simulink model "vehicleModel"  (R2023b)
settings: Solver=VariableStepAuto  StartTime=0.0  StopTime=10.0  RelTol=1e-3
values from neighbouring files (symbols this model uses):
  b1 = b(1,:)    [bicyclekinematicmodel.m]
  b2 = b(2,:)    [bicyclekinematicmodel.m]
undefined symbols (not defined in the file or in its folder): a, linear, position
libraries: ros2lib x8, fuzblock x1
settings Model: Creator=samee  LastModifiedBy=AUVSL

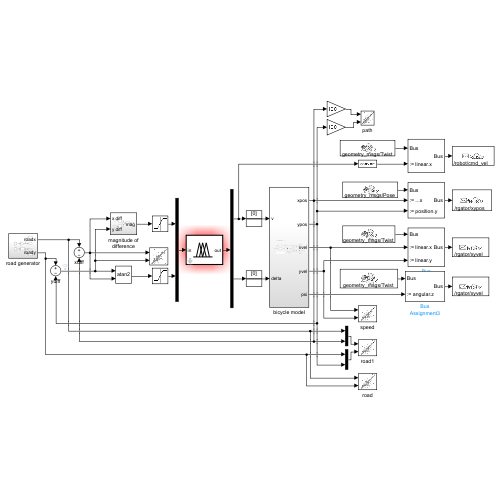
[thumbnail: Simulink's stored preview of the top-level diagram]
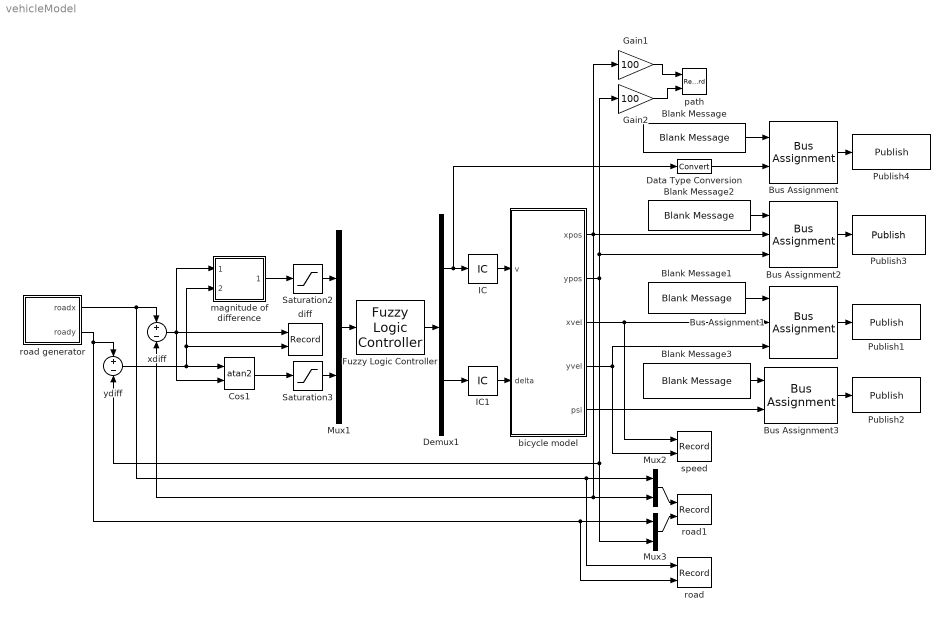
== system vehicleModel ==
  Blank Message : ros2lib/Blank Message  messageClass=Message  entityType=geometry_msgs/Twist  messageType=geometry_msgs/Twist  SampleTime=inf
  Blank Message1 : ros2lib/Blank Message  messageClass=Message  entityType=geometry_msgs/Twist  messageType=geometry_msgs/Twist  SampleTime=inf
  Blank Message2 : ros2lib/Blank Message  messageClass=Message  entityType=geometry_msgs/Pose  messageType=geometry_msgs/Pose  SampleTime=inf
  Blank Message3 : ros2lib/Blank Message  messageClass=Message  entityType=geometry_msgs/Twist  messageType=geometry_msgs/Twist  SampleTime=inf
  Bus Assignment : BusAssignment  AssignedSignals=linear.x
  Bus Assignment1 : BusAssignment  AssignedSignals=linear.x,linear.y
  Bus Assignment2 : BusAssignment  AssignedSignals=position.x,position.y
  Bus Assignment3 : BusAssignment  AssignedSignals=angular.z
  Cos1 : Trigonometry  Operator=atan2
  Data Type Conversion : DataTypeConversion  SaturateOnIntegerOverflow=off  RndMeth=Floor
  Demux1 : Demux  Outputs=2
  Fuzzy Logic Controller : fuzblock/Fuzzy Logic  Controller  FIS=fismatrix  OutputSampleNumber=101  DataType=double  FuzzifiedInputs=off  RuleFiringStrengths=off  RuleOutputs=off  AggregatedOutputs=off  SimulateUsing=Interpreted execution  OutOfRangeInputValueMessage=warning  NoRuleFiredMessage=warning  EmptyOutputFuzzySetMessage=warning
  Gain1 : Gain  Gain=100
  Gain2 : Gain  Gain=100
  IC : InitialCondition  Value=0
  IC1 : InitialCondition  Value=0
  Mux1 : Mux  Inputs=2
  Mux2 : Mux  Inputs=2
  Mux3 : Mux  Inputs=2
  Publish1 : ros2lib/Publish  topicSource=Specify your own  topic=/rgator/xyvel  messageType=geometry_msgs/Twist  QOSHistory=Keep last  QOSDepth=1  QOSReliability=Reliable  QOSDurability=Volatile
  Publish2 : ros2lib/Publish  topicSource=Specify your own  topic=/rgator/xyvel  messageType=geometry_msgs/Twist  QOSHistory=Keep last  QOSDepth=1  QOSReliability=Reliable  QOSDurability=Volatile
  Publish3 : ros2lib/Publish  topicSource=Specify your own  topic=/rgator/xypos  messageType=geometry_msgs/Pose  QOSHistory=Keep last  QOSDepth=1  QOSReliability=Reliable  QOSDurability=Volatile
  Publish4 : ros2lib/Publish  topicSource=Specify your own  topic=/robot/cmd_vel  messageType=geometry_msgs/Twist  QOSHistory=Keep last  QOSDepth=1  QOSReliability=Reliable  QOSDurability=Volatile
  Saturation2 : Saturate  UpperLimit=100  LowerLimit=0  LinearizeAsGain=off
  Saturation3 : Saturate  UpperLimit=1  LowerLimit=-1
  bicycle model : Subsystem
  diff : Record  FileSettingsInternal="{\"entries\":[{\"content\":{\"excelSettings\":{\"content\":{},\"type\":\"Streamout.ExcelSettings\"}},\"type\":\"Streamout.FileSettingStorage\",\"uuid\":\"\"}],\"packageUris\":[\"http:\\/\\/schema.mathworks.com\\/mf0\\/streamout_blocks\\/R2020a\"],\"version\":\"1.0\"}"  Layout=[1 1]  SignalsInternal="{\"entries\":[{\"content\":{\"signals\":[{\"content\":{\"blockPath\":[],\"dimensions\":[1],\"domain\":\"\",\"lineColor\":\"#edb120\",\"plots\":[ 1 ],\"port\":1,\"signalID\":1,\"signalName\":\"xdiff\"},\"type\":\"RecordBlkView.Signal\",\"uuid\":\"\"},{\"content\":{\"blockPath\":[],\"dimensions\":[1],\"domain\":\"\",\"lineColor\":\"#7e2f8e\",\"plots\":[ 1 ],\"port\":2,\"signalID\":2,\"signalName\":\"ydiff\"},\"type\":\"RecordBlkView.Signal\",\"uuid\":\"\"}]},\"type\":\"RecordBlkView.InputSignals\",\"uuid\":\"\"}],\"packageUris\":[\"http:\\/\\/schema.mathworks.com\\/mf0\\/streamout_blocks\\/R2020a\"],\"version\":\"1.0\"}"  VisualizationBindings="{\"xyplotplugin\":{\"info\":[{\"series\":[{\"bindingParametersList\":[{\"parameter\":\"X-Axis\",\"signalID\":1,\"signalName\":\"xdiff\"},{\"parameter\":\"Y-Axis\",\"signalID\":2,\"signalName\":\"ydiff\"}],\"seriesID\":0}],\"subplotID\":1}]}}"  CompatibilityTag=XY
  magnitude of difference : Subsystem
  path : Record  FileSettingsInternal="{\"entries\":[{\"content\":{\"excelSettings\":{\"content\":{},\"type\":\"Streamout.ExcelSettings\"}},\"type\":\"Streamout.FileSettingStorage\",\"uuid\":\"\"}],\"packageUris\":[\"http:\\/\\/schema.mathworks.com\\/mf0\\/streamout_blocks\\/R2020a\"],\"version\":\"1.0\"}"  Layout=[1 1]  SignalsInternal="{\"entries\":[{\"content\":{\"signals\":[{\"content\":{\"blockPath\":[],\"dimensions\":[1],\"domain\":\"\",\"lineColor\":\"#77ac30\",\"plots\":[ 1 ],\"port\":1,\"signalID\":1,\"signalName\":\"Gain\"},\"type\":\"RecordBlkView.Signal\",\"uuid\":\"\"},{\"content\":{\"blockPath\":[],\"dimensions\":[1],\"domain\":\"\",\"lineColor\":\"#4dbeee\",\"plots\":[ 1 ],\"port\":2,\"signalID\":2,\"signalName\":\"Gain1\"},\"type\":\"RecordBlkView.Signal\",\"uuid\":\"\"}]},\"type\":\"RecordBlkView.InputSignals\",\"uuid\":\"\"}],\"packageUris\":[\"http:\\/\\/schema.mathworks.com\\/mf0\\/streamout_blocks\\/R2020a\"],\"version\":\"1.0\"}"  VisualizationBindings="{\"xyplotplugin\":{\"info\":[{\"series\":[{\"bindingParametersList\":[{\"parameter\":\"X-Axis\",\"signalID\":1,\"signalName\":\"Gain\"},{\"parameter\":\"Y-Axis\",\"signalID\":2,\"signalName\":\"Gain1\"}],\"seriesID\":0}],\"subplotID\":1}]}}"  CompatibilityTag=XY
  road : Record  FileSettingsInternal="{\"entries\":[{\"content\":{\"excelSettings\":{\"content\":{},\"type\":\"Streamout.ExcelSettings\"}},\"type\":\"Streamout.FileSettingStorage\",\"uuid\":\"\"}],\"packageUris\":[\"http:\\/\\/schema.mathworks.com\\/mf0\\/streamout_blocks\\/R2020a\"],\"version\":\"1.0\"}"  Layout=[1 1]  SignalsInternal="{\"entries\":[{\"content\":{\"signals\":[{\"content\":{\"blockPath\":[],\"dimensions\":[1],\"domain\":\"\",\"lineColor\":\"#a2142f\",\"plots\":[ 1 ],\"port\":1,\"signalID\":1,\"signalName\":\"road generator:1\"},\"type\":\"RecordBlkView.Signal\",\"uuid\":\"\"},{\"content\":{\"blockPath\":[],\"dimensions\":[1],\"domain\":\"\",\"lineColor\":\"#139fff\",\"plots\":[ 1 ],\"port\":2,\"signalID\":2,\"signalName\":\"road generator:2\"},\"type\":\"RecordBlkView.Signal\",\"uuid\":\"\"}]},\"type\":\"RecordBlkView.InputSignals\",\"uuid\":\"\"}],\"packageUris\":[\"http:\\/\\/schema.mathworks.com\\/mf0\\/streamout_blocks\\/R2020a\"],\"version\":\"1.0\"}"  VisualizationBindings="{\"xyplotplugin\":{\"info\":[{\"series\":[{\"bindingParametersList\":[{\"parameter\":\"X-Axis\",\"signalID\":1,\"signalName\":\"road generator:1\"},{\"parameter\":\"Y-Axis\",\"signalID\":2,\"signalName\":\"road generator:2\"}],\"seriesID\":0}],\"subplotID\":1}]}}"  CompatibilityTag=XY
  road generator : Subsystem
  road1 : Record  FileSettingsInternal="{\"entries\":[{\"content\":{\"excelSettings\":{\"content\":{},\"type\":\"Streamout.ExcelSettings\"}},\"type\":\"Streamout.FileSettingStorage\",\"uuid\":\"\"}],\"packageUris\":[\"http:\\/\\/schema.mathworks.com\\/mf0\\/streamout_blocks\\/R2020a\"],\"version\":\"1.0\"}"  Layout=[1 1]  SignalsInternal="{\"entries\":[{\"content\":{\"signals\":[{\"content\":{\"blockPath\":[],\"dimensions\":[2],\"domain\":\"\",\"hasChildren\":true,\"lineColor\":\"#a2142f\",\"port\":1,\"signalID\":1,\"signalName\":\"Mux1\"},\"type\":\"RecordBlkView.Signal\",\"uuid\":\"\"},{\"content\":{\"blockPath\":[],\"channel\":[1],\"dimensions\":[2],\"domain\":\"\",\"lineColor\":\"#139fff\",\"parentID\":1,\"plots\":[ 1 ],\"port\":1,\"signalID\":2,\"signalName\":\"Mux1\"},\"type\":\"RecordBlkView.Signal\",\"uuid\":\"\"},{\"content\":{\"blockPath\":[],\"channel\":[2],\"dimensions\":[2],\"domain\":\"\",\"lineColor\":\"#fe330a\",\"parentID\":1,\"plots\":[ 1 ],\"port\":1,\"signalID\":3,\"signalName\":\"Mux1\"},\"type\":\"RecordBlkView.Signal\",\"uuid\":\"\"},{\"content\":{\"blockPath\":[],\"dimensions\":[2],\"domain\":\"\",\"hasChildren\":true,\"lineColor\":\"#ff6929\",\"port\":2,\"signalID\":4,\"signalName\":\"Mux2\"},\"type\":\"RecordBlkView.Signal\",\"uuid\":\"\"},{\"content\":{\"blockPath\":[],\"channel\":[1],\"dimensions\":[2],\"domain\":\"\",\"lineColor\":\"#b746ff\",\"parentID\":4,\"plots\":[ 1 ],\"port\":2,\"signalID\":5,\"signalName\":\"Mux2\"},\"type\":\"RecordBlkView.Signal\",\"uuid\":\"\"},{\"content\":{\"blockPath\":[],\"channel\":[2],\"dimensions\":[2],\"domain\":\"\",\"lineColor\":\"#22b573\",\"parentID\":4,\"plots\":[ 1 ],\"port\":2,\"signalID\":6,\"signalName\":\"Mux2\"},\"type\":\"RecordBlkView.Signal\",\"uuid\":\"\"}]},\"type\":\"RecordBlkView.InputSignals\",\"uuid\":\"\"}],\"packageUris\":[\"http:\\/\\/schema.mathworks.com\\/mf0\\/streamout_blocks\\/R2020a\"],\"version\":\"1.0\"}"  VisualizationBindings="{\"xyplotplugin\":{\"info\":[{\"series\":[{\"bindingParametersList\":[{\"parameter\":\"X-Axis\",\"signalID\":3,\"signalName\":\"Mux1(2)\"},{\"parameter\":\"Y-Axis\",\"signalID\":5,\"signalName\":\"Mux2(1)\"}],\"seriesID\":0},{\"bindingParametersList\":[{\"parameter\":\"X-Axis\",\"signalID\":2,\"signalName\":\"Mux1(1)\"},{\"parameter\":\"Y-Axis\",\"signalID\":6,\"signalName\":\"Mux2(2)\"}],\"seriesID\":1}],\"subplotID\":1}]}}"  CompatibilityTag=XY
  speed : Record  FileSettingsInternal="{\"entries\":[{\"content\":{\"excelSettings\":{\"content\":{},\"type\":\"Streamout.ExcelSettings\"}},\"type\":\"Streamout.FileSettingStorage\",\"uuid\":\"\"}],\"packageUris\":[\"http:\\/\\/schema.mathworks.com\\/mf0\\/streamout_blocks\\/R2020a\"],\"version\":\"1.0\"}"  Layout=[1 1]  SignalsInternal="{\"entries\":[{\"content\":{\"signals\":[{\"content\":{\"blockPath\":[],\"dimensions\":[1],\"domain\":\"\",\"lineColor\":\"#ff6929\",\"plots\":[ 1 ],\"port\":1,\"signalID\":1,\"signalName\":\"bicycle model:3\"},\"type\":\"RecordBlkView.Signal\",\"uuid\":\"\"},{\"content\":{\"blockPath\":[],\"dimensions\":[1],\"domain\":\"\",\"lineColor\":\"#b746ff\",\"plots\":[ 1 ],\"port\":2,\"signalID\":2,\"signalName\":\"bicycle model:4\"},\"type\":\"RecordBlkView.Signal\",\"uuid\":\"\"}]},\"type\":\"RecordBlkView.InputSignals\",\"uuid\":\"\"}],\"packageUris\":[\"http:\\/\\/schema.mathworks.com\\/mf0\\/streamout_blocks\\/R2020a\"],\"version\":\"1.0\"}"  VisualizationBindings="{\"xyplotplugin\":{\"info\":[{\"series\":[{\"bindingParametersList\":[{\"parameter\":\"X-Axis\",\"signalID\":1,\"signalName\":\"bicycle model:3\"},{\"parameter\":\"Y-Axis\",\"signalID\":2,\"signalName\":\"bicycle model:4\"}],\"seriesID\":0}],\"subplotID\":1}]}}"  CompatibilityTag=XY
  xdiff : Sum  Inputs=+-
  ydiff : Sum  Inputs=+-
  wires:
  Mux2/1 -> road1/1
  Saturation2/1 -> Mux1/1
  Fuzzy Logic Controller/1 -> Demux1/1
  Demux1/2 -> IC1/1
  ydiff/1 -> magnitude of difference/2(y diff), diff/2, Cos1/1
  Mux1/1 -> Fuzzy Logic Controller/1
  road generator/2(roady) -> road/2, Mux3/1, ydiff/1
  Blank Message1/1 -> Bus Assignment1/1
  Blank Message/1 -> Bus Assignment/1
  Bus Assignment3/1 -> Publish2/1
  Blank Message3/1 -> Bus Assignment3/1
  Bus Assignment2/1 -> Publish3/1
  road generator/1(roadx) -> xdiff/1, Mux2/1, road/1
  Demux1/1 -> Data Type Conversion/1, IC/1
  Bus Assignment1/1 -> Publish1/1
  bicycle model/5(psi) -> Bus Assignment3/2
  IC1/1 -> bicycle model/2(delta)
  magnitude of difference/1(mag) -> Saturation2/1
  Saturation3/1 -> Mux1/2
  bicycle model/3(xvel) -> speed/1, Bus Assignment1/2
  Gain2/1 -> path/2
  bicycle model/1(xpos) -> Gain1/1, xdiff/2, Mux2/2, Bus Assignment2/2
  Cos1/1 -> Saturation3/1
  xdiff/1 -> Cos1/2, diff/1, magnitude of difference/1(x diff)
  IC/1 -> bicycle model/1(v)
  Mux3/1 -> road1/2
  Gain1/1 -> path/1
  Bus Assignment/1 -> Publish4/1
  bicycle model/4(yvel) -> Bus Assignment1/3, speed/2
  bicycle model/2(ypos) -> Gain2/1, Bus Assignment2/3, Mux3/2, ydiff/2
  Blank Message2/1 -> Bus Assignment2/1
  Data Type Conversion/1 -> Bus Assignment/2

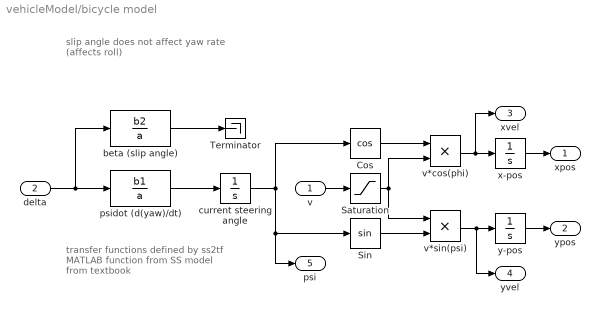
== system vehicleModel/bicycle model ==
  note: transfer functions defined by ss2tf
      | MATLAB function from SS model
      | from textbook
  note: slip angle does not affect yaw rate
      | (affects roll)
  v : Inport
  delta : Inport  Port=2  OutDataTypeStr=double
  Cos : Trigonometry  Operator=cos
  Saturation : Saturate  UpperLimit=30  LowerLimit=-30
  Sin : Trigonometry
  Terminator : Terminator
  beta (slip angle) : TransferFcn  Numerator=b2  Denominator=a  ContinuousStateAttributes='beta'
  current steering angle : Integrator
  psidot (d(yaw)/dt) : TransferFcn  Numerator=b1  Denominator=a  ParameterTunability=Optimized  ContinuousStateAttributes='psidot'
  v*cos(phi) : Product
  v*sin(psi) : Product
  x-pos : Integrator
  y-pos : Integrator
  xpos : Outport
  ypos : Outport  Port=2
  xvel : Outport  Port=3
  yvel : Outport  Port=4
  psi : Outport  Port=5
  wires:
  psidot (d(yaw)/dt)/1 -> current steering angle/1
  v*sin(psi)/1 -> y-pos/1, yvel/1
  current steering angle/1 -> psi/1, Sin/1, Cos/1
  delta/1 -> psidot (d(yaw)/dt)/1, beta (slip angle)/1
  Sin/1 -> v*sin(psi)/2
  v*cos(phi)/1 -> x-pos/1, xvel/1
  Cos/1 -> v*cos(phi)/1
  y-pos/1 -> ypos/1
  x-pos/1 -> xpos/1
  Saturation/1 -> v*cos(phi)/2, v*sin(psi)/1
  v/1 -> Saturation/1
  beta (slip angle)/1 -> Terminator/1

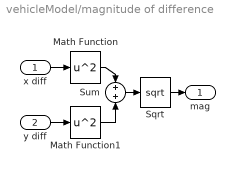
== system vehicleModel/magnitude of difference ==
  x diff : Inport
  y diff : Inport  Port=2
  Math Function : Math  Operator=square
  Math Function1 : Math  Operator=square
  Sqrt : Sqrt
  Sum : Sum  Inputs=+|+
  mag : Outport
  wires:
  Math Function/1 -> Sum/1
  Sum/1 -> Sqrt/1
  Math Function1/1 -> Sum/2
  y diff/1 -> Math Function1/1
  Sqrt/1 -> mag/1
  x diff/1 -> Math Function/1

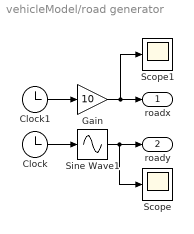
== system vehicleModel/road generator ==
  Clock : Clock
  Clock1 : Clock
  Gain : Gain  Gain=10
  Scope : Scope
  Scope1 : Scope
  Sine Wave1 : Sin  TimeSource=Use external signal  Amplitude=10  Frequency=0.05  Phase=1  SampleTime=0
  roadx : Outport
  roady : Outport  Port=2
  wires:
  Clock/1 -> Sine Wave1/1
  Sine Wave1/1 -> Scope/1, roady/1
  Clock1/1 -> Gain/1
  Gain/1 -> roadx/1, Scope1/1
